simulink model "aircraft"  (R2024a)
settings: Solver=VariableStepAuto  StartTime=0.0  StopTime=inf  RelTol=1e-3
libraries: instrumentseriallib x3, svdutilitieslib x2
settings Model: Creator=ADMIN  LastModifiedBy=ADMIN

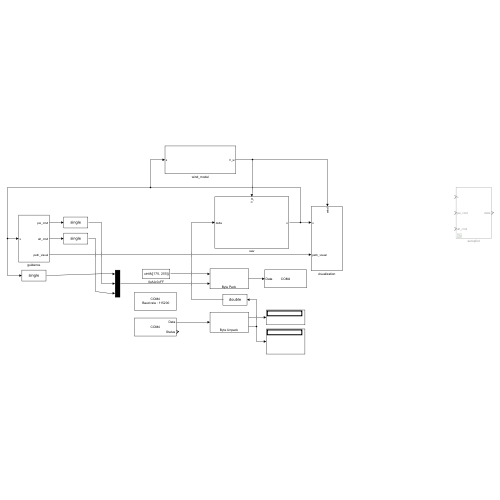
[thumbnail: Simulink's stored preview of the top-level diagram]
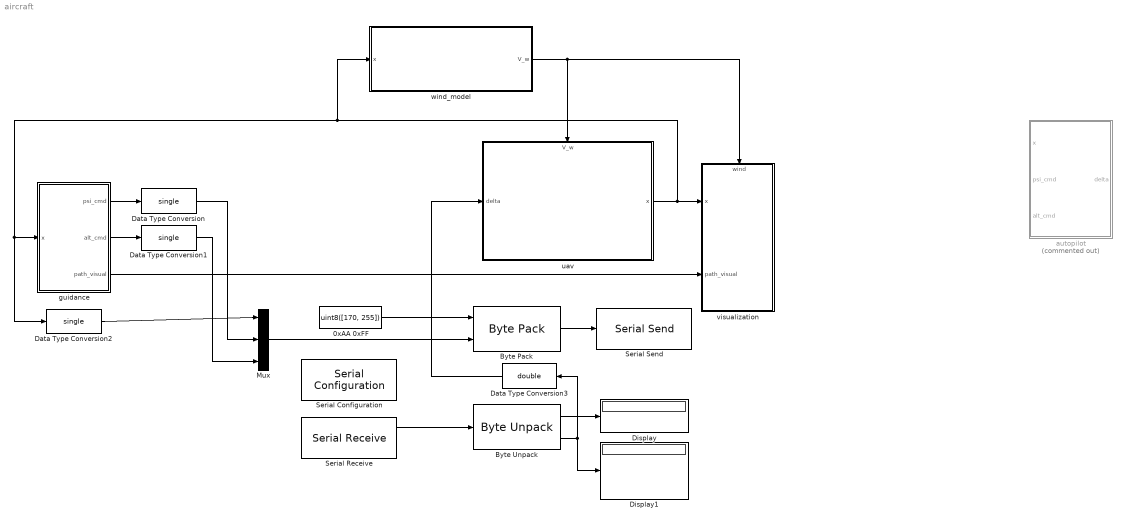
== system aircraft ==
  0xAA 0xFF : Constant  Value=uint8([170, 255])
  Byte Pack : svdutilitieslib/Byte Pack  maskPackedDataType=uint8  datatypes={'uint8', 'single'}  byteAlign=1  blockPlatform=tic2000
      settings: LibrarySourceBlock=c2000lib/Target Communication/Byte Pack
  Byte Unpack : svdutilitieslib/Byte Unpack  dimensions={[2] [4]}  datatypes={'uint8', 'single'}  byteAlign=1  blockPlatform=tic2000
      settings: LibrarySourceBlock=c2000lib/Target Communication/Byte Unpack
  Data Type Conversion : DataTypeConversion  OutDataTypeStr=single  SaturateOnIntegerOverflow=off  RndMeth=Floor
  Data Type Conversion1 : DataTypeConversion  OutDataTypeStr=single  SaturateOnIntegerOverflow=off  RndMeth=Floor
  Data Type Conversion2 : DataTypeConversion  OutDataTypeStr=single  SaturateOnIntegerOverflow=off  RndMeth=Floor
  Data Type Conversion3 : DataTypeConversion  OutDataTypeStr=double  SaturateOnIntegerOverflow=off  RndMeth=Floor
  Display : Display
  Display1 : Display
  Mux : Mux  Inputs=3
  Serial Configuration : instrumentseriallib/Serial Configuration  Priority=-200000  PortSel=COM4  Port=COM4  ComPort=COM4  BaudRate=115200  DataBits=8  Parity=none  StopBits=1  ByteOrder=little-endian  FlowControl=none  Timeout=10  SimulateUsing=Interpreted execution  BlockInModel=on  aMode=1
  Serial Receive : instrumentseriallib/Serial Receive  Priority=1  PortSel=COM4  Port=COM4  ComPort=COM4  DataType=uint8  SaveDataType=uint8  ToggleHeader=off  Header=[]  ToggleDataSize=on  DataSize=[18 1]  ToggleTerminator=off  Terminator=<none>  CustomTerminator=[]  InputFormat=Column major  EnableBlockingMode=off  ActionDataUnavailable=Output last received value  ActionWhenDataUnavailable=Output last received value  CustomValue=0  SampleTime=0.01  SimulateUsing=Interpreted execution  BlockInModel=on  aMode=1
      settings: LibrarySourceBlock=c2000lib/Host Communication/Serial Receive
  Serial Send : instrumentseriallib/Serial Send  Priority=1  PortSel=COM4  Port=COM4  ComPort=COM4  Header=[]  Terminator=<none>  CustomTerminator=[]  EnableBlockingMode=off  SimulateUsing=Interpreted execution  BlockInModel=on  aMode=1
      settings: LibrarySourceBlock=c2000lib/Host Communication/Serial Send
  "autopilot " : Subsystem  Commented=on
  guidance : Subsystem
  "uav " : Subsystem
      settings: PortSchema="{\"entries\":[{\"content\":{\"sides\":[{\"content\":{\"connectorIds\":[\"In1\"]},\"type\":\"ConnectorPlacement.EquallySpacedRectSide\",\"uuid\":\"a7b46c76-63bb-4654-bcb2-91627cecb901\"},{\"content\":{\"connectorIds\":[\"Out1\"],\"side\":\"RIGHT\"},\"type\":\"ConnectorPlacement.EquallySpacedRectSide\",\"uuid\":\"e45597e5-281a-43ae-9b8f-01f809ae90a8\"},{\"content\":{\"connectorIds\":[\"In2\"],\"side\":\"TOP\"},\"type\":\"ConnectorPlacement.EquallySpacedRectSide\",\"uuid\":\"e4f93d17-0834-49b6-953c-d959a9d487bc\"}]},\"type\":\"ConnectorPlacement.EquallySpacedConnector\",\"uuid\":\"aee35d44-0504-4876-b308-b0d63ae44a1f\"}],\"packageUris\":[\"http://schema.mathworks.com/mf0/Connector/R2020b\"],\"version\":\"1.0\"}"
  visualization : Subsystem
      settings: PortSchema="{\"entries\":[{\"content\":{\"sides\":[{\"content\":{\"connectorIds\":[\"In1\",\"In2\"]},\"type\":\"ConnectorPlacement.EquallySpacedRectSide\",\"uuid\":\"3ca85e6b-5690-4cee-b297-0410b8eb8b03\"},{\"content\":{\"side\":\"RIGHT\"},\"type\":\"ConnectorPlacement.EquallySpacedRectSide\",\"uuid\":\"b077d845-b4f0-4046-b1ae-a0ce879f315b\"},{\"content\":{\"connectorIds\":[\"In3\"],\"side\":\"TOP\"},\"type\":\"ConnectorPlacement.EquallySpacedRectSide\",\"uuid\":\"5282982d-07cb-4dd6-a7f3-d3fc714f27f8\"}]},\"type\":\"ConnectorPlacement.EquallySpacedConnector\",\"uuid\":\"6eccf57b-fb72-419b-a501-32d6f52412a8\"}],\"packageUris\":[\"http://schema.mathworks.com/mf0/Connector/R2020b\"],\"version\":\"1.0\"}"
  wind_model : Subsystem
  wires:
  "uav "/1(x) -> wind_model/1(x), Data Type Conversion2/1, guidance/1(x), visualization/1(x)
  guidance/3(path_visual) -> visualization/2(path_visual)
  wind_model/1(V_w) -> "uav "/2(V_w), visualization/3(wind)
  Byte Unpack/1 -> Display/1
  Serial Receive/1 -> Byte Unpack/1
  Byte Unpack/2 -> Data Type Conversion3/1, Display1/1
  Byte Pack/1 -> Serial Send/1
  0xAA 0xFF/1 -> Byte Pack/1
  Mux/1 -> Byte Pack/2
  guidance/1(psi_cmd) -> Data Type Conversion/1
  guidance/2(alt_cmd) -> Data Type Conversion1/1
  Data Type Conversion2/1 -> Mux/1
  Data Type Conversion/1 -> Mux/2
  Data Type Conversion1/1 -> Mux/3
  Data Type Conversion3/1 -> "uav "/1(delta)

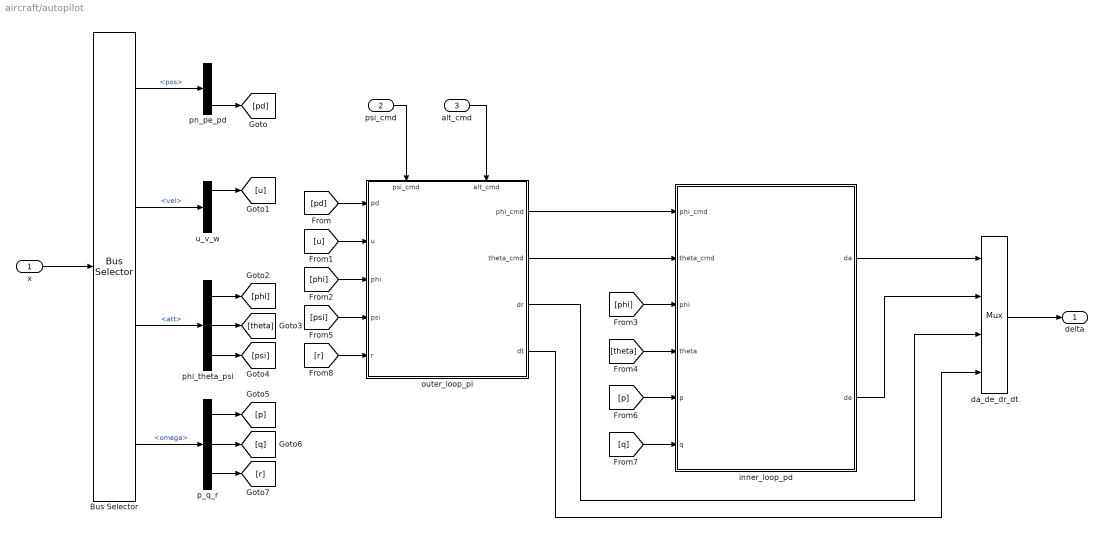
== system aircraft/autopilot  ==
  x : Inport
  psi_cmd : Inport  Port=2
  alt_cmd : Inport  Port=3
  Bus Selector : BusSelector  OutputSignals=pos,vel,att,omega
  da_de_dr_dt : Mux
  inner_loop_pd : Subsystem
  outer_loop_pi : Subsystem
      settings: PortSchema="{\"entries\":[{\"content\":{\"sides\":[{\"content\":{\"connectorIds\":[\"In1\",\"In2\",\"In3\",\"In4\",\"In5\"]},\"type\":\"ConnectorPlacement.EquallySpacedRectSide\",\"uuid\":\"f8b93ce5-1209-4743-a4f6-40947377afa0\"},{\"content\":{\"connectorIds\":[\"Out1\",\"Out2\",\"Out3\",\"Out4\"],\"side\":\"RIGHT\"},\"type\":\"ConnectorPlacement.EquallySpacedRectSide\",\"uuid\":\"38b86da4-8ea0-4db2-a7be-1fc292de95ff\"},{\"content\":{\"connectorIds\":[\"In6\",\"In7\"],\"side\":\"TOP\"},\"type\":\"ConnectorPlacement.EquallySpacedRectSide\",\"uuid\":\"879dde49-1a12-4f2d-a7d9-4a8a8e5f8381\"}]},\"type\":\"ConnectorPlacement.EquallySpacedConnector\",\"uuid\":\"28f217f5-b437-4f7c-874d-3ab28b03532d\"}],\"packageUris\":[\"http://schema.mathworks.com/mf0/Connector/R2020b\"],\"version\":\"1.0\"}"
  p_q_r : Demux  Outputs=3
  phi_theta_psi : Demux  Outputs=3
  pn_pe_pd : Demux  Outputs=3
  u_v_w : Demux  Outputs=3
  delta : Outport
  wires:
  da_de_dr_dt/1 -> delta/1
  Bus Selector/3 -> phi_theta_psi/1  "<att>"
  Bus Selector/4 -> p_q_r/1  "<omega>"
  Bus Selector/1 -> pn_pe_pd/1  "<pos>"
  Bus Selector/2 -> u_v_w/1  "<vel>"
  inner_loop_pd/1(da) -> da_de_dr_dt/1
  inner_loop_pd/2(de) -> da_de_dr_dt/2
  outer_loop_pi/1(phi_cmd) -> inner_loop_pd/1(phi_cmd)
  outer_loop_pi/2(theta_cmd) -> inner_loop_pd/2(theta_cmd)
  outer_loop_pi/3(dr) -> da_de_dr_dt/3
  outer_loop_pi/4(dt) -> da_de_dr_dt/4
  pn_pe_pd/3 -> [pd]
  [pd] -> outer_loop_pi/1(pd)
  u_v_w/1 -> [u]
  [u] -> outer_loop_pi/2(u)
  phi_theta_psi/1 -> [phi]
  [phi] -> outer_loop_pi/3(phi)
  [phi] -> inner_loop_pd/3(phi)
  phi_theta_psi/2 -> [theta]
  [theta] -> inner_loop_pd/4(theta)
  phi_theta_psi/3 -> [psi]
  [psi] -> outer_loop_pi/4(psi)
  p_q_r/1 -> [p]
  p_q_r/2 -> [q]
  [p] -> inner_loop_pd/5(p)
  [q] -> inner_loop_pd/6(q)
  p_q_r/3 -> [r]
  [r] -> outer_loop_pi/5(r)
  psi_cmd/1 -> outer_loop_pi/6(psi_cmd)
  alt_cmd/1 -> outer_loop_pi/7(alt_cmd)
  x/1 -> Bus Selector/1

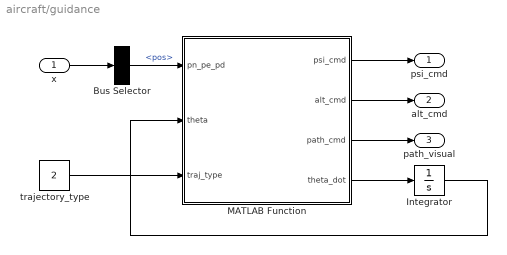
== system aircraft/guidance ==
  x : Inport
  Bus Selector : BusSelector  OutputSignals=pos
  Integrator : Integrator
  MATLAB Function : MATLAB Function  TreatAsAtomicUnit=on
  trajectory_type : Constant  Value=2
  psi_cmd : Outport
  alt_cmd : Outport  Port=2
  path_visual : Outport  Port=3
  wires:
  trajectory_type/1 -> MATLAB Function/3(traj_type)
  Integrator/1 -> MATLAB Function/2(theta)
  MATLAB Function/1(psi_cmd) -> psi_cmd/1
  MATLAB Function/2(alt_cmd) -> alt_cmd/1
  MATLAB Function/3(path_cmd) -> path_visual/1
  MATLAB Function/4(theta_dot) -> Integrator/1
  x/1 -> Bus Selector/1
  Bus Selector/1 -> MATLAB Function/1(pn_pe_pd)  "<pos>"

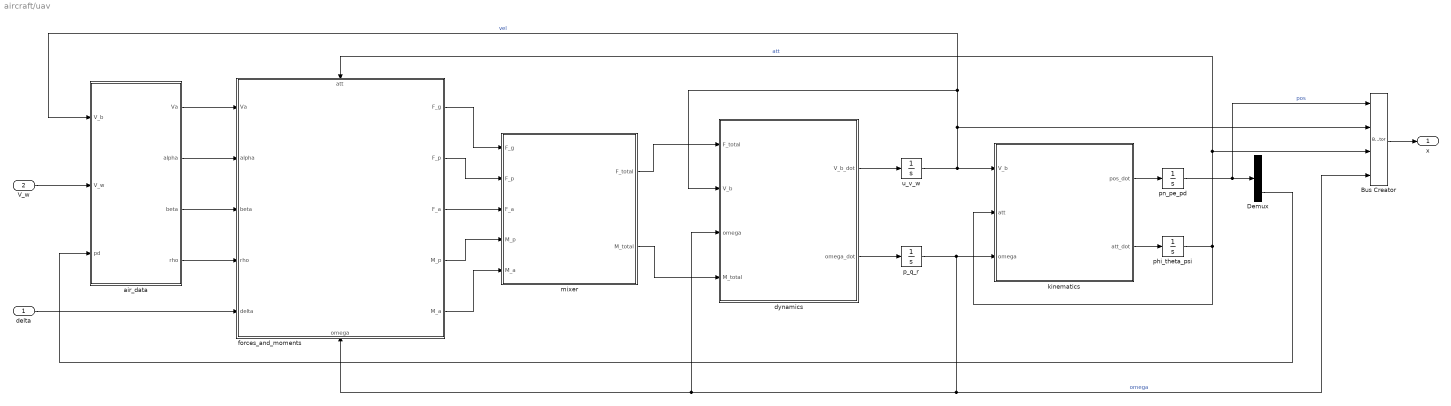
== system aircraft/uav  ==
  delta : Inport
  V_w : Inport  Port=2
  Bus Creator : BusCreator  Inputs=4
  Demux : Demux  Outputs=3
  air_data : MATLAB Function  TreatAsAtomicUnit=on
  dynamics : Subsystem
  forces_and_moments : Subsystem
      settings: PortSchema="{\"entries\":[{\"content\":{\"sides\":[{\"content\":{\"connectorIds\":[\"In1\",\"In2\",\"In3\",\"In4\",\"In5\"]},\"type\":\"ConnectorPlacement.EquallySpacedRectSide\",\"uuid\":\"faed5ae1-1da7-4bdb-9f91-d07bb241893e\"},{\"content\":{\"connectorIds\":[\"Out1\",\"Out2\",\"Out3\",\"Out4\",\"Out5\"],\"side\":\"RIGHT\"},\"type\":\"ConnectorPlacement.EquallySpacedRectSide\",\"uuid\":\"3869cb38-1eed-4d47-9855-45677924a456\"},{\"content\":{\"connectorIds\":[\"In6\"],\"side\":\"TOP\"},\"type\":\"ConnectorPlacement.EquallySpacedRectSide\",\"uuid\":\"bdf63fef-403e-488a-a985-bca31845462f\"},{\"content\":{\"connectorIds\":[\"In7\"],\"side\":\"BOTTOM\"},\"type\":\"ConnectorPlacement.EquallySpacedRectSide\",\"uuid\":\"22a16173-6ad3-41e9-b567-c24186f01d1d\"}]},\"type\":\"ConnectorPlacement.EquallySpacedConnector\",\"uuid\":\"20fa0166-ef5c-40dd-8a30-826f9f2a65f7\"}],\"packageUris\":[\"http://schema.mathworks.com/mf0/Connector/R2020b\"],\"version\":\"1.0\"}"
  kinematics : Subsystem
  mixer : MATLAB Function  TreatAsAtomicUnit=on
  p_q_r : Integrator  InitialCondition=[0; 0; 0]
  phi_theta_psi : Integrator  InitialCondition=[0; 0.14622; 0]
  pn_pe_pd : Integrator  InitialCondition=[0; 0; -100]
  u_v_w : Integrator  InitialCondition=[15; 0; 3.3029]
  x : Outport
  wires:
  p_q_r/1 -> Bus Creator/4, dynamics/3(omega), forces_and_moments/7(omega), kinematics/3(omega)  "omega"
  kinematics/2(att_dot) -> phi_theta_psi/1
  u_v_w/1 -> kinematics/1(V_b), Bus Creator/2, air_data/1(V_b), dynamics/2(V_b)  "vel"
  pn_pe_pd/1 -> Bus Creator/1, Demux/1  "pos"
  dynamics/1(V_b_dot) -> u_v_w/1
  air_data/1(Va) -> forces_and_moments/1(Va)
  phi_theta_psi/1 -> Bus Creator/3, forces_and_moments/6(att), kinematics/2(att)  "att"
  forces_and_moments/2(F_p) -> mixer/2(F_p)
  kinematics/1(pos_dot) -> pn_pe_pd/1
  forces_and_moments/3(F_a) -> mixer/3(F_a)
  Bus Creator/1 -> x/1
  mixer/1(F_total) -> dynamics/1(F_total)
  mixer/2(M_total) -> dynamics/4(M_total)
  V_w/1 -> air_data/2(V_w)
  air_data/2(alpha) -> forces_and_moments/2(alpha)
  air_data/3(beta) -> forces_and_moments/3(beta)
  forces_and_moments/1(F_g) -> mixer/1(F_g)
  forces_and_moments/4(M_p) -> mixer/4(M_p)
  air_data/4(rho) -> forces_and_moments/4(rho)
  forces_and_moments/5(M_a) -> mixer/5(M_a)
  Demux/3 -> air_data/3(pd)
  dynamics/2(omega_dot) -> p_q_r/1
  delta/1 -> forces_and_moments/5(delta)

== system aircraft/visualization ==
  x : Inport
  path_visual : Inport  Port=2
  wind : Inport  Port=3
  Bus Selector : BusSelector  OutputSignals=att,pos
  MATLAB Function : MATLAB Function  TreatAsAtomicUnit=on
  wind_visualization : Scope
  wires:
  path_visual/1 -> MATLAB Function/3(path_cmd)
  x/1 -> Bus Selector/1
  Bus Selector/2 -> MATLAB Function/1(pn_pe_pd)  "<pos>"
  Bus Selector/1 -> MATLAB Function/2(phi_theta_psi)  "<att>"
  wind/1 -> wind_visualization/1

== system aircraft/wind_model ==
  x : Inport
  Bus Selector : BusSelector  OutputSignals=att
  Constant : Constant  Value=[2; 4; 1]
  MATLAB Function : MATLAB Function  TreatAsAtomicUnit=on
  V_w : Outport
  wires:
  x/1 -> Bus Selector/1
  Bus Selector/1 -> MATLAB Function/1(phi_theta_psi)  "<att>"
  Constant/1 -> MATLAB Function/2(Vw_inertial)
  MATLAB Function/1(Vw_body) -> V_w/1

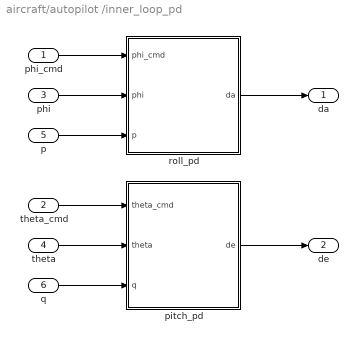
== system aircraft/autopilot /inner_loop_pd ==
  phi_cmd : Inport
  theta_cmd : Inport  Port=2
  phi : Inport  Port=3
  theta : Inport  Port=4
  p : Inport  Port=5
  q : Inport  Port=6
  pitch_pd : Subsystem
  roll_pd : Subsystem
  da : Outport
  de : Outport  Port=2
  wires:
  phi/1 -> roll_pd/2(phi)
  theta_cmd/1 -> pitch_pd/1(theta_cmd)
  theta/1 -> pitch_pd/2(theta)
  q/1 -> pitch_pd/3(q)
  p/1 -> roll_pd/3(p)
  pitch_pd/1(de) -> de/1
  roll_pd/1(da) -> da/1
  phi_cmd/1 -> roll_pd/1(phi_cmd)

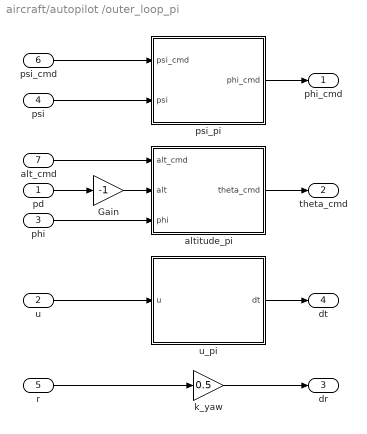
== system aircraft/autopilot /outer_loop_pi ==
  pd : Inport
  u : Inport  Port=2
  phi : Inport  Port=3
  psi : Inport  Port=4
  r : Inport  Port=5
  psi_cmd : Inport  Port=6
  alt_cmd : Inport  Port=7
  Gain : Gain  Gain=-1
  altitude_pi : Subsystem
  k_yaw : Gain  Gain=0.5
  psi_pi : Subsystem
  u_pi : Subsystem
  phi_cmd : Outport
  theta_cmd : Outport  Port=2
  dr : Outport  Port=3
  dt : Outport  Port=4
  wires:
  Gain/1 -> altitude_pi/2(alt)
  pd/1 -> Gain/1
  phi/1 -> altitude_pi/3(phi)
  psi/1 -> psi_pi/2(psi)
  altitude_pi/1(theta_cmd) -> theta_cmd/1
  u/1 -> u_pi/1(u)
  k_yaw/1 -> dr/1
  psi_pi/1(phi_cmd) -> phi_cmd/1
  u_pi/1(dt) -> dt/1
  r/1 -> k_yaw/1
  psi_cmd/1 -> psi_pi/1(psi_cmd)
  alt_cmd/1 -> altitude_pi/1(alt_cmd)

== system aircraft/uav /dynamics ==
  F_total : Inport
  V_b : Inport  Port=2
  omega : Inport  Port=3
  M_total : Inport  Port=4
  rotational_dynamics : MATLAB Function  TreatAsAtomicUnit=on
  translational_dynamics : MATLAB Function  TreatAsAtomicUnit=on
  V_b_dot : Outport
  omega_dot : Outport  Port=2
  wires:
  omega/1 -> translational_dynamics/3(omega), rotational_dynamics/2(omega)
  M_total/1 -> rotational_dynamics/1(M_total)
  translational_dynamics/1(V_b_dot) -> V_b_dot/1
  rotational_dynamics/1(omega_dot) -> omega_dot/1
  V_b/1 -> translational_dynamics/2(V_b)
  F_total/1 -> translational_dynamics/1(F_total)

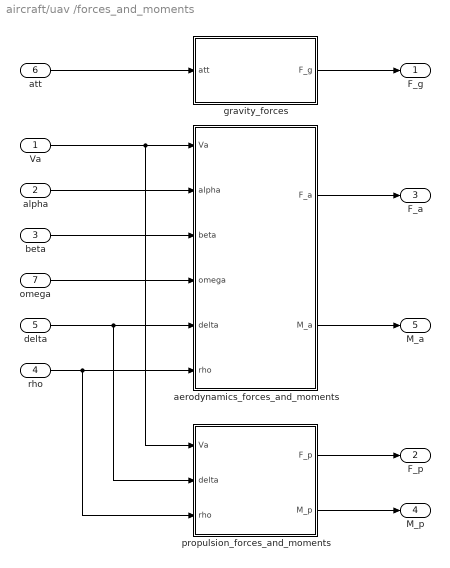
== system aircraft/uav /forces_and_moments ==
  Va : Inport
  alpha : Inport  Port=2
  beta : Inport  Port=3
  rho : Inport  Port=4
  delta : Inport  Port=5
  att : Inport  Port=6
  omega : Inport  Port=7
  aerodynamics_forces_and_moments : MATLAB Function  TreatAsAtomicUnit=on
  gravity_forces : MATLAB Function  TreatAsAtomicUnit=on
  propulsion_forces_and_moments : MATLAB Function  TreatAsAtomicUnit=on
  F_g : Outport
  F_p : Outport  Port=2
  F_a : Outport  Port=3
  M_p : Outport  Port=4
  M_a : Outport  Port=5
  wires:
  beta/1 -> aerodynamics_forces_and_moments/3(beta)
  rho/1 -> propulsion_forces_and_moments/3(rho), aerodynamics_forces_and_moments/6(rho)
  att/1 -> gravity_forces/1(att)
  Va/1 -> propulsion_forces_and_moments/1(Va), aerodynamics_forces_and_moments/1(Va)
  alpha/1 -> aerodynamics_forces_and_moments/2(alpha)
  propulsion_forces_and_moments/1(F_p) -> F_p/1
  omega/1 -> aerodynamics_forces_and_moments/4(omega)
  propulsion_forces_and_moments/2(M_p) -> M_p/1
  aerodynamics_forces_and_moments/2(M_a) -> M_a/1
  aerodynamics_forces_and_moments/1(F_a) -> F_a/1
  gravity_forces/1(F_g) -> F_g/1
  delta/1 -> propulsion_forces_and_moments/2(delta), aerodynamics_forces_and_moments/5(delta)

== system aircraft/uav /kinematics ==
  V_b : Inport
  att : Inport  Port=2
  omega : Inport  Port=3
  rotational_kinematics : MATLAB Function  TreatAsAtomicUnit=on
  translational_kinematics : MATLAB Function  TreatAsAtomicUnit=on
  pos_dot : Outport
  att_dot : Outport  Port=2
  wires:
  translational_kinematics/1(pos_dot) -> pos_dot/1
  omega/1 -> rotational_kinematics/1(omega)
  att/1 -> rotational_kinematics/2(att), translational_kinematics/2(att)
  rotational_kinematics/1(att_dot) -> att_dot/1
  V_b/1 -> translational_kinematics/1(V_b)

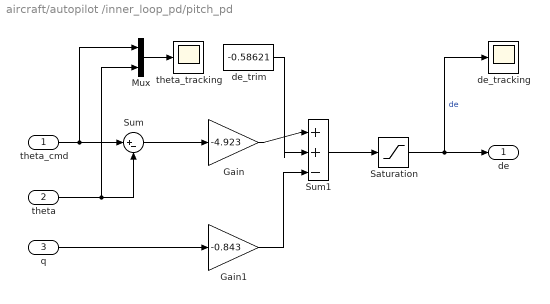
== system aircraft/autopilot /inner_loop_pd/pitch_pd ==
  theta_cmd : Inport
  theta : Inport  Port=2
  q : Inport  Port=3
  Gain : Gain  Gain=-4.923
  Gain1 : Gain  Gain=-0.843
  Mux : Mux  Inputs=2
  Saturation : Saturate  UpperLimit=1  LowerLimit=-1
  Sum : Sum  Inputs=|+-
  Sum1 : Sum  Inputs=|++-
  de_tracking : Scope
  de_trim : Constant  Value=-0.58621
  theta_tracking : Scope
  de : Outport
  wires:
  Saturation/1 -> de_tracking/1, de/1  "de"
  Sum1/1 -> Saturation/1
  q/1 -> Gain1/1
  Sum/1 -> Gain/1
  theta_cmd/1 -> Mux/1, Sum/1
  theta/1 -> Mux/2, Sum/2
  Mux/1 -> theta_tracking/1
  Gain/1 -> Sum1/1
  Gain1/1 -> Sum1/3
  de_trim/1 -> Sum1/2

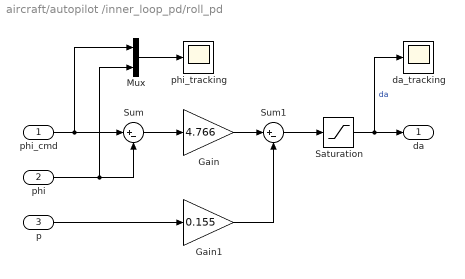
== system aircraft/autopilot /inner_loop_pd/roll_pd ==
  phi_cmd : Inport
  phi : Inport  Port=2
  p : Inport  Port=3
  Gain : Gain  Gain=4.766
  Gain1 : Gain  Gain=0.155
  Mux : Mux  Inputs=2
  Saturation : Saturate  UpperLimit=0.436  LowerLimit=-0.436
  Sum : Sum  Inputs=|+-
  Sum1 : Sum  Inputs=|+-
  da_tracking : Scope
  phi_tracking : Scope
  da : Outport
  wires:
  Gain1/1 -> Sum1/2
  phi/1 -> Sum/2, Mux/2
  Sum/1 -> Gain/1
  p/1 -> Gain1/1
  phi_cmd/1 -> Mux/1, Sum/1
  Sum1/1 -> Saturation/1
  Saturation/1 -> da_tracking/1, da/1  "da"
  Mux/1 -> phi_tracking/1
  Gain/1 -> Sum1/1

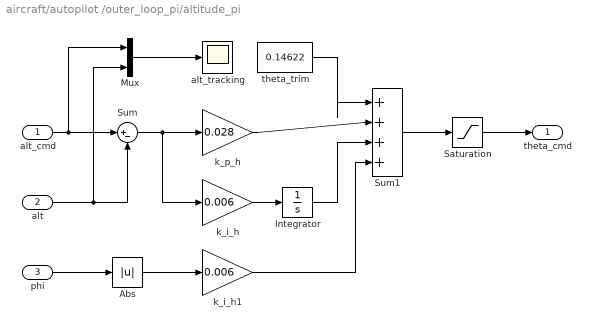
== system aircraft/autopilot /outer_loop_pi/altitude_pi ==
  alt_cmd : Inport
  alt : Inport  Port=2
  phi : Inport  Port=3
  Abs : Abs  SaturateOnIntegerOverflow=off
  Integrator : Integrator  LimitOutput=on  UpperSaturationLimit=0.261  LowerSaturationLimit=-0.261
  Mux : Mux  Inputs=2
  Saturation : Saturate  UpperLimit=0.7  LowerLimit=-0.7
  Sum : Sum  Inputs=|+-
  Sum1 : Sum  Inputs=|++++
  alt_tracking : Scope
  k_i_h : Gain  Gain=0.006
  k_i_h1 : Gain  Gain=0.006
  k_p_h : Gain  Gain=0.028
  theta_trim : Constant  Value=0.14622
  theta_cmd : Outport
  wires:
  Mux/1 -> alt_tracking/1
  Saturation/1 -> theta_cmd/1
  Sum1/1 -> Saturation/1
  alt_cmd/1 -> Sum/1, Mux/1
  Sum/1 -> k_i_h/1, k_p_h/1
  alt/1 -> Mux/2, Sum/2
  k_i_h/1 -> Integrator/1
  Integrator/1 -> Sum1/3
  k_p_h/1 -> Sum1/2
  theta_trim/1 -> Sum1/1
  phi/1 -> Abs/1
  Abs/1 -> k_i_h1/1
  k_i_h1/1 -> Sum1/4

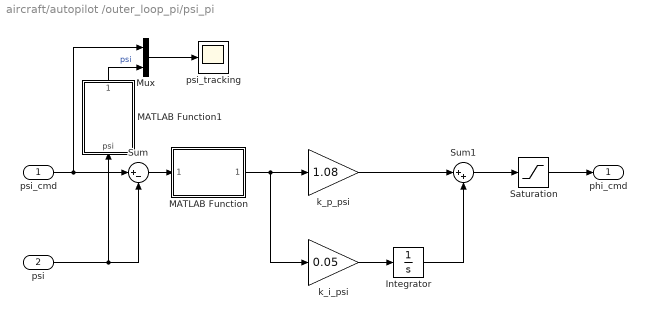
== system aircraft/autopilot /outer_loop_pi/psi_pi ==
  psi_cmd : Inport
  psi : Inport  Port=2
  Integrator : Integrator  LimitOutput=on  UpperSaturationLimit=0.436  LowerSaturationLimit=-0.436
  MATLAB Function : MATLAB Function  TreatAsAtomicUnit=on
  MATLAB Function1 : MATLAB Function  TreatAsAtomicUnit=on
  Mux : Mux  Inputs=2
  Saturation : Saturate  UpperLimit=0.436  LowerLimit=-0.436
  Sum : Sum  Inputs=|+-
  Sum1 : Sum  Inputs=|++
  k_i_psi : Gain  Gain=0.05
  k_p_psi : Gain  Gain=1.08
  psi_tracking : Scope
  phi_cmd : Outport
  wires:
  Integrator/1 -> Sum1/2
  k_i_psi/1 -> Integrator/1
  psi/1 -> Sum/2, MATLAB Function1/1(psi)
  Sum/1 -> MATLAB Function/1(error_in)
  Sum1/1 -> Saturation/1
  Saturation/1 -> phi_cmd/1
  Mux/1 -> psi_tracking/1
  k_p_psi/1 -> Sum1/1
  MATLAB Function/1(error_out) -> k_i_psi/1, k_p_psi/1
  psi_cmd/1 -> Mux/1, Sum/1
  MATLAB Function1/1(psi_wrapped) -> Mux/2  "psi"

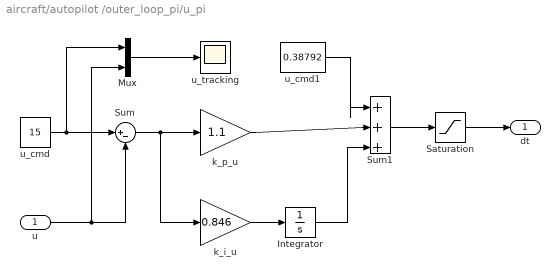
== system aircraft/autopilot /outer_loop_pi/u_pi ==
  u : Inport
  Integrator : Integrator  LimitOutput=on  UpperSaturationLimit=1  LowerSaturationLimit=0
  Mux : Mux  Inputs=2
  Saturation : Saturate  UpperLimit=1  LowerLimit=0
  Sum : Sum  Inputs=|+-
  Sum1 : Sum  Inputs=|+++
  k_i_u : Gain  Gain=0.846
  k_p_u : Gain  Gain=1.1
  u_cmd : Constant  Value=15
  u_cmd1 : Constant  Value=0.38792
  u_tracking : Scope
  dt : Outport
  wires:
  k_p_u/1 -> Sum1/2
  Mux/1 -> u_tracking/1
  Saturation/1 -> dt/1
  Sum1/1 -> Saturation/1
  u_cmd/1 -> Sum/1, Mux/1
  Sum/1 -> k_i_u/1, k_p_u/1
  u/1 -> Mux/2, Sum/2
  k_i_u/1 -> Integrator/1
  Integrator/1 -> Sum1/3
  u_cmd1/1 -> Sum1/1

== matlab function aircraft/uav /kinematics/translational_kinematics ==
  data: V_b input; pos_dot output size=[3, 1]; att input
function pos_dot = trans_kinematics(V_b, att)
    % inputs:
    %   V_b:     [3x1] body velocities [u; v; w] (m/s)
    %   att:     [3x1] euler angles [phi; theta; psi] (rad)
    % outputs:
    %   pos_dot: [3x1] inertial pos derivatives [pn_dot; pe_dot; pd_dot] (m/s)

    u = V_b(1); v = V_b(2); w = V_b(3);
    phi = att(1); theta = att(2); psi = att(3);

    cphi = cos(phi); sphi = sin(phi);
    cthe = cos(theta); sthe = sin(theta);
    cpsi = cos(psi); spsi = sin(psi);

    R_b_v = [cthe*cpsi, sphi*sthe*cpsi - cphi*spsi, cphi*sthe*cpsi + sphi*spsi;
             cthe*spsi, sphi*sthe*spsi + cphi*cpsi, cphi*sthe*spsi - sphi*cpsi;
             -sthe,     sphi*cthe,                  cphi*cthe];
             
    pos_dot = R_b_v * [u; v; w];
end

== matlab function aircraft/autopilot /outer_loop_pi/psi_pi/MATLAB Function ==
  data: error_in input; error_out output
function error_out = wrap_angle(error_in)
    % wraps any angle to strictly [-pi, pi]
    error_out = mod(error_in + pi, 2*pi) - pi;
end

== matlab function aircraft/visualization/MATLAB Function ==
  data: pn_pe_pd input; phi_theta_psi input; path_cmd input
function draw_uav_3d(pn_pe_pd, phi_theta_psi, path_cmd)
    coder.extrinsic('update_uav_plot');
    update_uav_plot(pn_pe_pd, phi_theta_psi, path_cmd);
end

== matlab function aircraft/guidance/MATLAB Function ==
  data: pn_pe_pd input; psi_cmd output size=[1, 1]; theta input; traj_type input; alt_cmd output; path_cmd output size=[4, 1]; theta_dot output size=[1, 1]
function [psi_cmd, alt_cmd, path_cmd, theta_dot] = generate_trajectory(pn_pe_pd, theta, traj_type)
    % Extract current UAV position
    pn = pn_pe_pd(1);
    pe = pn_pe_pd(2);
    
    A = 300;
    V_uav = 15.0; 
    N_center = 500;
    E_center = 500;
    
    if traj_type == 1
        % --- 1. FIGURE-8 (Lemniscate) ---
        % theta represents the CARROT's current position
        N_carrot = N_center + A * sin(theta) * cos(theta);
        E_carrot = E_center + A * sin(theta);
        Alt_carrot = 100;
        
        % Calculate path gradients at the carrot
        dN_dtheta = A * cos(2 * theta);
        dE_dtheta = A * cos(theta);
        
    else
        % --- 2. HELIX (Climbing Circle) ---
        N_carrot = N_center + A * cos(theta);
        E_carrot = E_center + A * sin(theta);
        Alt_carrot = 100 + (13.0 * theta); 
        
        dN_dtheta = -A * sin(theta);
        dE_dtheta = A * cos(theta);
    end
    
    % --- THE VIRTUAL TARGET FEEDBACK LOOP ---
    % 1. Calculate actual physical distance between UAV and Carrot
    d_actual = sqrt((N_carrot - pn)^2 + (E_carrot - pe)^2);
    
    % 2. Enforce a strict Lookahead Tether (e.g., exactly 40 meters)
    L_desired = 40.0;
    
    % 3. Carrot Speed Controller: 
    % If d_actual < 40, carrot speeds up. If d_actual > 40, it slows down.
    k_carrot = 1.5; % Tuning gain for target speed
    V_carrot = V_uav + k_carrot * (L_desired - d_actual);
    % --- SATURATION: Prevent supersonic carrot speeds ---
    if V_carrot > 25.0
        V_carrot = 25.0; % Max sprint speed
    elseif V_carrot < 0.0
        V_carrot = 0.0;  % Stop and wait for UAV
    end
    
    % 4. Convert linear carrot speed to angular geometric speed
    gradient = sqrt(dN_dtheta^2 + dE_dtheta^2);
    theta_dot = V_carrot / gradient;
    
    % --- THE GUIDANCE LAW ---
    chi_los = atan2(E_carrot - pe, N_carrot - pn);
    chi_q = atan2(dE_dtheta, dN_dtheta);
    
    error_los = mod((chi_los - chi_q) + pi, 2*pi) - pi;
    
    % Heading Command = Path Tangent + Proportional Correction
    k_path = 1.2; 
    psi_cmd = chi_q + (k_path * error_los);
    
    alt_cmd = Alt_carrot;
    
    % Output for 3D visualizer
    path_cmd = [N_carrot; E_carrot; Alt_carrot; traj_type];
end

== matlab function aircraft/wind_model/MATLAB Function ==
  data: phi_theta_psi input; Vw_body output; Vw_inertial input
function Vw_body = rotate_wind(phi_theta_psi, Vw_inertial)
    phi = phi_theta_psi(1);
    theta = phi_theta_psi(2);
    psi = phi_theta_psi(3);

    % Rotation Matrix from Inertial to Body Frame (R_v^b)
    R_yaw = [cos(psi), sin(psi), 0; -sin(psi), cos(psi), 0; 0, 0, 1];
    R_pitch = [cos(theta), 0, -sin(theta); 0, 1, 0; sin(theta), 0, cos(theta)];
    R_roll = [1, 0, 0; 0, cos(phi), sin(phi); 0, -sin(phi), cos(phi)];
    
    R_v_to_b = R_roll * R_pitch * R_yaw;
    
    % Total body frame wind (Ready for gusts to be added later)
    Vw_body = R_v_to_b * Vw_inertial;
end

== matlab function aircraft/autopilot /outer_loop_pi/psi_pi/MATLAB Function1 ==
  data: psi input; psi_wrapped output
function psi_wrapped = wrap_plot(psi)
    psi_wrapped = mod(psi + pi, 2*pi) - pi;
end

== matlab function aircraft/uav /forces_and_moments/gravity_forces ==
  data: att input; F_g output; P parameter
function F_g = calculate_gravity(att, P)
    % inputs:
    %   att:  [3x1] euler angles [phi; theta; psi] (rad)
    %   mass: [1x1] uav mass (kg)
    %   g:    [1x1] gravitational constant (m/s^2)
    % outputs:
    %   F_g:  [3x1] gravity forces [fx; fy; fz] (n)
    
    phi   = att(1);
    theta = att(2);
    
    % project gravity to body frame
    F_g = P.mass * P.g * [-sin(theta);
                           cos(theta) * sin(phi);
                           cos(theta) * cos(phi)];
end

== matlab function aircraft/uav /air_data ==
  data: V_b input; Va output; V_w input; pd input; alpha output; beta output; rho output; P parameter
function [Va, alpha, beta, rho] = calculate_env_data(V_b, V_w, pd, P)
    % inputs:
    %   V_b: [3x1] body-frame ground velocity [u; v; w] (m/s)
    %   V_w: [3x1] body-frame wind velocity [uw; vw; ww] (m/s)
    %   pd:  [1x1] down position (negative of altitude) (m)
    % outputs:
    %   Va:     [1x1] airspeed magnitude (m/s)
    %   alpha:  [1x1] angle of attack (rad)
    %   beta:   [1x1] sideslip angle (rad)
    
    % current height
    h = -pd;
    
    % temperature and pressure at altitude h
    T = P.T0 + P.L0 * h;
    p = P.p0 * (P.T0 / T)^((P.g * P.Molar) / (P.R * P.L0));
    
    % dynamic density using ideal gas law
    rho = (p * P.Molar) / (P.R * T);
    
    % airspeed vector
    V_r = V_b - V_w;
    
    % airspeed magnitude
    Va = norm(V_r);
    
    % angle of attack and sideslip
    if Va == 0 % prevent to divide by zero
        alpha = 0;
        beta  = 0;
    else
        alpha = atan2(V_r(3), V_r(1));
        beta  = asin(V_r(2) / Va);
    end
end

== matlab function aircraft/uav /forces_and_moments/aerodynamics_forces_and_moments ==
  data: Va input; F_a output; alpha input; beta input; M_a output; omega input; delta input size=[4, 1]; rho input; P parameter
function [F_a, M_a] = calculate_aerodynamics(Va, alpha, beta, ...
                                             omega, delta, rho, P)
    % inputs:
    %   Va:    [1x1] airspeed (m/s)
    %   alpha: [1x1] angle of attack (rad)
    %   beta:  [1x1] sideslip angle (rad)
    %   omega: [3x1] body angular rates [p; q; r] (rad/s)
    %   delta: [4x1] control signals [da; de; dr; dt]
    %   rho:   [1x1] air density (kg/m^3)
    %   P:     [1x1 struct] aerodynamic parameters
    % outputs:
    %   F_a:   [3x1] aerodynamic forces [fax; fay; faz] (n)
    %   M_a:   [3x1] aerodynamic moments [max; may; maz] (n-m)
    
    p = omega(1);
    q = omega(2);
    r = omega(3);
    
    da = delta(1);
    de = delta(2);
    dr = delta(3);
    
    % prevent division by zero at rest
    if Va == 0
        F_a = [0; 0; 0];
        M_a = [0; 0; 0];
        return;
    end
    
    % sigmoid blending function for non-linear stall
    sig_num = 1 + exp(-P.M * (alpha - P.alpha0)) + ...
        exp(P.M * (alpha + P.alpha0));
    sig_den = (1 + exp(-P.M * (alpha - P.alpha0))) * ...
        (1 + exp(P.M * (alpha + P.alpha0)));
    sigma_alpha = sig_num / sig_den;
    
    % non-linear lift coefficient
    CL_linear = P.C_L0 + P.C_Lalpha * alpha;
    CL_flat   = 2 * sign(alpha) * sin(alpha)^2 * cos(alpha);
    CL_alpha  = (1 - sigma_alpha) * CL_linear + sigma_alpha * CL_flat;
    
    % non-linear drag coefficient (quadratic)
    AR = (P.b^2) / P.S;
    CD_alpha = P.C_D0 + (CL_linear^2) / (pi * P.e * AR);
    
    % longitudinal aerodynamic coefficients
    cx      = -CD_alpha * cos(alpha) + CL_alpha * sin(alpha);
    cx_q    = -P.C_Dq * cos(alpha) + P.C_Lq * sin(alpha);
    cx_de   = -P.C_Dde * cos(alpha) + P.C_Lde * sin(alpha);
    
    cz      = -CD_alpha * sin(alpha) - CL_alpha * cos(alpha);
    cz_q    = -P.C_Dq * sin(alpha) - P.C_Lq * cos(alpha);
    cz_de   = -P.C_Dde * sin(alpha) - P.C_Lde * cos(alpha);
    
    % dynamic pressure terms
    q_bar = 0.5 * rho * Va^2 * P.S;
    c_2v  = (P.c * q) / (2 * Va);
    b_2v_p = (P.b * p) / (2 * Va);
    b_2v_r = (P.b * r) / (2 * Va);
    
    % compute forces
    fax = q_bar * (cx + cx_q * c_2v + cx_de * de);
    fay = q_bar * (P.C_Y0 + P.C_Ybeta * beta + P.C_Yp * b_2v_p + ...
        P.C_Yr * b_2v_r + P.C_Yda * da + P.C_Ydr * dr);
    faz = q_bar * (cz + cz_q * c_2v + cz_de * de);
    
    % compute moments
    max = q_bar * P.b * (P.C_Mx0 + P.C_Mxbeta * beta + ...
        P.C_Mxp * b_2v_p + P.C_Mxr * b_2v_r + ...
        P.C_Mxda * da + P.C_Mxdr * dr);
    may = q_bar * P.c * (P.C_My0 + P.C_Myalpha * alpha + ...
        P.C_Myq * c_2v + P.C_Myde * de);
    maz = q_bar * P.b * (P.C_Mz0 + P.C_Mzbeta * beta + ...
        P.C_Mzp * b_2v_p + P.C_Mzr * b_2v_r + ...
        P.C_Mzda * da + P.C_Mzdr * dr);
    
    F_a = [fax; fay; faz];
    M_a = [max; may; maz];
end

== matlab function aircraft/uav /forces_and_moments/propulsion_forces_and_moments ==
  data: Va input; F_p output; delta input; M_p output; rho input; P parameter
function [F_p, M_p] = calculate_propulsion(Va, delta, rho, P)
    % calculates propulsion forces and moments[cite: 1]
    % inputs:
    %   Va:   [1x1] airspeed (m/s)
    %   delta:[4x1] control signals [da; de; dr; dt]
    %   rho:  [1x1] air density (kg/m^3)
    %   P:    [1x1 struct] physical parameters
    % outputs:
    %   F_p:  [3x1] propulsive force [fx; fy; fz] (n)
    %   M_p:  [3x1] propulsive moment [mx; my; mz] (n-m)

    dt = delta(4);
    if dt == 0
        F_p = [0; 0; 0];
        M_p = [0; 0; 0];
        return;
    end
    
    v_in = P.V_max * dt;
    
    a = (rho * P.D_prop^5) / ((2 * pi)^2) * P.C_Q0;
    b = (rho * P.D_prop^4) / (2 * pi) * P.C_Q1 * Va + ...
        (P.k_Q * P.k_V) / P.R_motor;
    c = rho * P.D_prop^3 * P.C_Q2 * Va^2 - ...
        (P.k_Q / P.R_motor) * v_in + P.k_Q * P.i0;
    
    omega_p = (-b + sqrt(b^2 - 4 * a * c)) / (2 * a);
    
    t_p = (rho * P.D_prop^4) / ((2 * pi)^2) * omega_p^2 * P.C_T0 + ...
          (rho * P.D_prop^3) / (2 * pi) * omega_p * Va * P.C_T1 + ...
          rho * P.D_prop^2 * Va^2 * P.C_T2;
          
    q_p = (rho * P.D_prop^5) / ((2 * pi)^2) * omega_p^2 * P.C_Q0 + ...
          (rho * P.D_prop^4) / (2 * pi) * omega_p * Va * P.C_Q1 + ...
          rho * P.D_prop^3 * Va^2 * P.C_Q2;
          
    F_p = [t_p; 0; 0];
    M_p = [-q_p; 0; 0];
end

== matlab function aircraft/uav /mixer ==
  data: F_g input; F_total output; F_p input; F_a input; M_p input; M_a input; M_total output
function [F_total, M_total] = mix_forces_moments(F_g, F_p, F_a, M_p, M_a)
    % sums all forces and moments[cite: 1]
    % inputs:
    %   F_g: [3x1] gravity force (n)
    %   F_p: [3x1] propulsive force (n)
    %   F_a: [3x1] aerodynamic force (n)
    %   M_p: [3x1] propulsive moment (n-m)
    %   M_a: [3x1] aerodynamic moment (n-m)
    % outputs:
    %   F_total: [3x1] total body frame force (n)
    %   M_total: [3x1] total body frame moment (n-m)

    F_total = F_g + F_p + F_a;
    M_total = M_p + M_a;
end

== matlab function aircraft/uav /dynamics/translational_dynamics ==
  data: F_total input; V_b input; V_b_dot output size=[3, 1]; omega input; P parameter
function V_b_dot = trans_dynamics(F_total, V_b, omega, P)
    % inputs:
    %   F_total: [3x1] total forces [fx; fy; fz] (n)
    %   V_b:     [3x1] body velocities [u; v; w] (m/s)
    %   omega:   [3x1] angular rates [p; q; r] (rad/s)
    %   P:       [1x1 struct] physical parameters
    % outputs:
    %   V_b_dot: [3x1] velocity derivatives [u_dot; v_dot; w_dot] (m/s^2)

    u = V_b(1); v = V_b(2); w = V_b(3);
    p = omega(1); q = omega(2); r = omega(3);
    fx = F_total(1); 
    fy = F_total(2); 
    fz = F_total(3);

    u_dot = r*v - q*w + fx / P.mass;
    v_dot = p*w - r*u + fy / P.mass;
    w_dot = q*u - p*v + fz / P.mass;
    
    V_b_dot = [u_dot; v_dot; w_dot];
end

== matlab function aircraft/uav /dynamics/rotational_dynamics ==
  data: M_total input; omega_dot output size=[3, 1]; omega input; P parameter
function omega_dot = rot_dynamics(M_total, omega, P)
    % inputs:
    %   M_total:   [3x1] total moments [mx; my; mz] (n-m)
    %   omega:     [3x1] angular rates [p; q; r] (rad/s)
    %   P:         [1x1 struct] physical parameters
    % outputs:
    %   omega_dot: [3x1] angular rate derivatives [p_dot; q_dot; r_dot] (rad/s^2)

    p = omega(1); q = omega(2); r = omega(3);
    mx = M_total(1); my = M_total(2); mz = M_total(3);

    p_dot = P.Gamma1*p*q - P.Gamma2*q*r + P.Gamma3*mx + P.Gamma4*mz;
    q_dot = P.Gamma5*p*r - P.Gamma6*(p^2 - r^2) + my / P.Jy;
    r_dot = P.Gamma7*p*q - P.Gamma1*q*r + P.Gamma4*mx + P.Gamma8*mz;
    
    omega_dot = [p_dot; q_dot; r_dot];
end

== matlab function aircraft/uav /kinematics/rotational_kinematics ==
  data: omega input; att_dot output size=[3, 1]; att input
function att_dot = rot_kinematics(omega, att)
    % inputs:
    %   omega:   [3x1] angular rates [p; q; r] (rad/s)
    %   att:     [3x1] euler angles [phi; theta; psi] (rad)
    % outputs:
    %   att_dot: [3x1] euler angle derivatives [phi_dot; theta_dot; psi_dot] (rad/s)

    p = omega(1); q = omega(2); r = omega(3);
    phi = att(1); theta = att(2);

    cphi = cos(phi); sphi = sin(phi);
    cthe = cos(theta); tthe = tan(theta);

    R_rot = [1, sphi*tthe, cphi*tthe;
             0, cphi,      -sphi;
             0, sphi/cthe, cphi/cthe];
             
    att_dot = R_rot * [p; q; r];
end
